simulink subsystem "PieroControladoVPIz"  (R2025a)
settings: Solver=VariableStepAuto  StartTime=0.0  StopTime=10.0  RelTol=1e-3
settings Model: Creator=Antonio  LastModifiedBy=aj
settings RTWCC: GPUComputeCapability=3.5

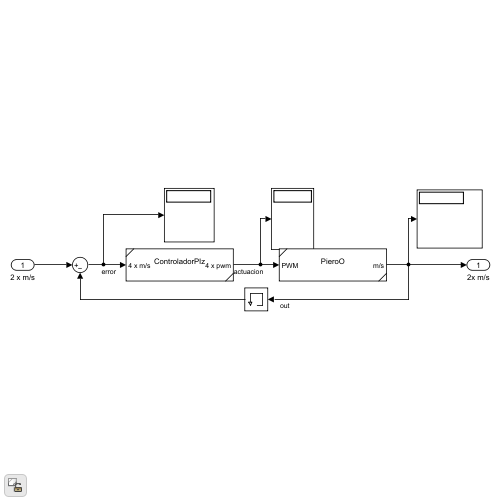
[thumbnail: Simulink's stored preview of the top-level diagram]
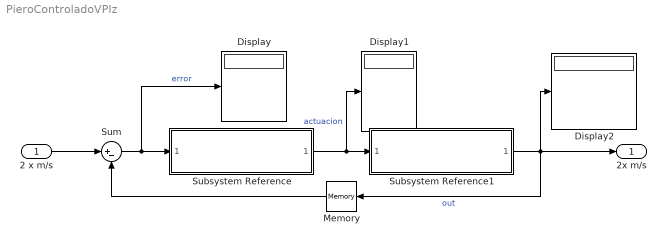
== system PieroControladoVPIz ==
  2 x m/s : Inport
  Display : Display
  Display1 : Display
  Display2 : Display
  Memory : Memory
  Subsystem Reference : Subsystem  ReferencedSubsystem=ControladorPIz
  Subsystem Reference1 : Subsystem  ReferencedSubsystem=PieroO
  Sum : Sum  Inputs=|+-
  2x m/s : Outport
  wires:
  Memory/1 -> Sum/2
  Subsystem Reference1/1 -> 2x m/s/1, Memory/1, Display2/1  "out"
  Sum/1 -> Display/1, Subsystem Reference/1  "error"
  2 x m/s/1 -> Sum/1
  Subsystem Reference/1 -> Display1/1, Subsystem Reference1/1  "actuacion"
